simulink model "dcom_project"  (R2024b)
settings: Solver=VariableStepAuto  StartTime=0.0  StopTime=10.0  RelTol=1e-3
libraries: simulink x8, dspquant2 x8, dspfdesign x4, dspsigops x4, commdigbbndam3 x2
settings Model: Creator=HP  LastModifiedBy=HP

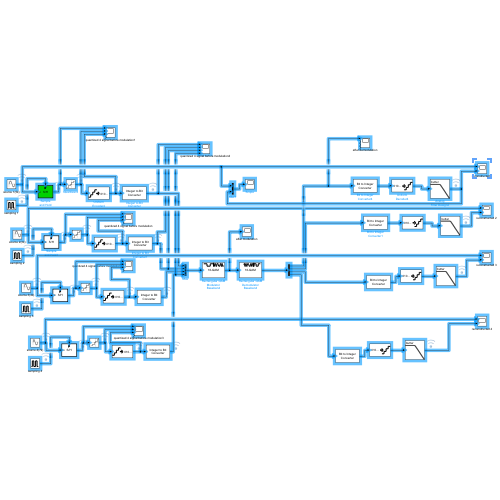
[thumbnail: Simulink's stored preview of the top-level diagram]
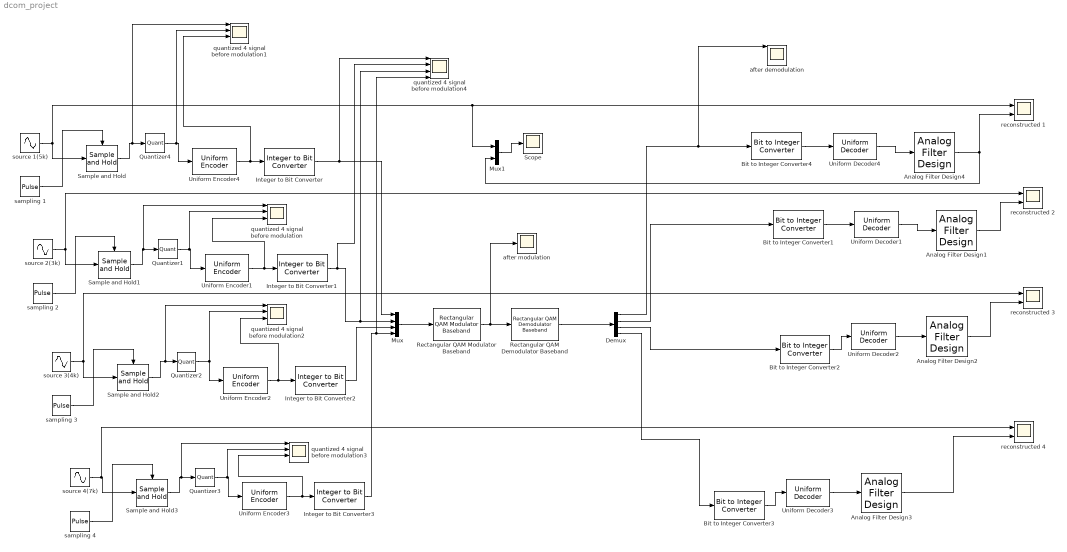
== system dcom_project ==
  Analog Filter Design1 : dspfdesign/Analog Filter Design  method=Butterworth  filttype=Lowpass  N=8  Wlo=2*pi*3000  Whi=80  Rp=2  Rs=40
  Analog Filter Design2 : dspfdesign/Analog Filter Design  method=Butterworth  filttype=Lowpass  N=8  Wlo=2*pi*4000  Whi=80  Rp=2  Rs=40
  Analog Filter Design3 : dspfdesign/Analog Filter Design  method=Butterworth  filttype=Lowpass  N=8  Wlo=2*pi*7000  Whi=80  Rp=2  Rs=40
  Analog Filter Design4 : dspfdesign/Analog Filter Design  method=Butterworth  filttype=Lowpass  N=8  Wlo=2*pi*5000  Whi=80  Rp=2  Rs=40
  Bit to Integer Converter{1..4} (4 alike) : simulink/Logic and Bit Operations/Bit to Integer Converter  nbits=4  bitOrder=MSB first  signedOutputValues=Signed  outDtype=Inherit via internal rule  outDtypeSigned=int8
      settings: LibrarySourceBlock=|
      | commutil2/Bit to Integer
      | Converter
  Demux : Demux
  Integer to Bit Converter{,1..3} (4 alike) : simulink/Logic and Bit Operations/Integer to Bit Converter  nbits=4  signedInputValues=Signed  bitOrder=MSB first  outDtype=Inherit via internal rule
      settings: LibrarySourceBlock=|
      | commutil2/Integer to Bit
      | Converter
  Mux : Mux
  Mux1 : Mux  Inputs=2
  Quantizer{1..4} (4 alike) : Quantizer  QuantizationInterval=0.125
  Rectangular QAM Demodulator Baseband : commdigbbndam3/Rectangular QAM Demodulator Baseband  M=16  OutType=Bit  DecType=Hard decision  VarSource=Dialog  Variance=1  Dec=Gray  Mapping=[0:15]  PowType=Min. distance between symbols  MinDist=2  AvgPow=1  PeakPow=1  Ph=0  outDtype1=Inherit via internal rule  outDtype2=Inherit via internal rule  derotateFactorWordLen=16  derotateFactorDataTypeStr=Inherit: Same word length as input  derotateFactorLastDataTypeStr=Inherit: Same word length as input  denormFactorWordLen=16  denormFactorDataTypeStr=Inherit: Same word length as input  denormFactorLastDataTypeStr=Inherit: Same word length as input  prodOutWordLen=32  prodOutOverflowMode=Wrap  prodOutRoundingMode=Floor  prodOutOvFlMode=off  prodOutOvFlModeLastStrValue=off  sumWordLen=32
      settings: LibrarySourceBlock=|
      | commhdldigbbndam/Rectangular QAM
      | Demodulator
      | Baseband
  Rectangular QAM Modulator Baseband : commdigbbndam3/Rectangular QAM Modulator Baseband  M=16  InType=Bit  Enc=Gray  Mapping=[0:15]  PowType=Min. distance between symbols  MinDist=2  AvgPow=1  PeakPow=1  Ph=0  outDtype=double  outWordLen=16  outUDDataType=sfix(16)  outFracLenMode=Best precision  outFracLen=15  outDataTypeStr=double  outLastDataTypeStr=double
      settings: LibrarySourceBlock=|
      | commhdldigbbndam/Rectangular QAM
      | Modulator
      | Baseband
  Sample and Hold{,1..3} (4 alike) : dspsigops/Sample and Hold  trig=Rising edge  initCond=0  latchinput=off
  Scope : Scope
  Uniform Decoder1 : dspquant2/Uniform Decoder  peak=5  bits=4  overflowMode=Saturate  otype=double
  Uniform Decoder2 : dspquant2/Uniform Decoder  peak=5  bits=4  overflowMode=Saturate  otype=double
  Uniform Decoder3 : dspquant2/Uniform Decoder  peak=5  bits=4  overflowMode=Saturate  otype=double
  Uniform Decoder4 : dspquant2/Uniform Decoder  peak=1.5  bits=4  overflowMode=Saturate  otype=double
  Uniform Encoder{1..4} (4 alike) : dspquant2/Uniform Encoder  peak=1.5  bits=4  otype=Signed integer
  after demodulation : Scope  NumInputPorts=4
  after modulation : Scope
  quantized 4 signal before modulation{,1..4} (5 alike) : Scope  NumInputPorts=4
  reconstructed {1..4} (4 alike) : Scope  NumInputPorts=2
  sampling 1 : DiscretePulseGenerator  PulseType=Time based  Period=1/40000  PulseWidth=50
  sampling 2 : DiscretePulseGenerator  PulseType=Time based  Period=1/24000  PulseWidth=50
  sampling 3 : DiscretePulseGenerator  PulseType=Time based  Period=1/32000  PulseWidth=50
  sampling 4 : DiscretePulseGenerator  PulseType=Time based  Period=1/56000  PulseWidth=50
  source 1(5k) : Sin  Frequency=2*pi*5000  Phase=pi/2  SampleTime=0
  source 2(3k) : Sin  Frequency=2*pi*3000  Phase=pi/2  SampleTime=0
  source 3(4k) : Sin  Frequency=2*pi*4000  Phase=pi/2  SampleTime=0
  source 4(7k) : Sin  Frequency=2*pi*7000  Phase=pi/2  SampleTime=0
  wires:
  sampling 1/1 -> Sample and Hold/Trigger
  Sample and Hold/1 -> quantized 4 signal before modulation1/1, Quantizer4/1
  Quantizer4/1 -> quantized 4 signal before modulation1/2, Uniform Encoder4/1
  Uniform Encoder4/1 -> quantized 4 signal before modulation1/3, Integer to Bit Converter/1
  Sample and Hold1/1 -> quantized 4 signal before modulation/1, Quantizer1/1
  Uniform Encoder1/1 -> quantized 4 signal before modulation/3, Integer to Bit Converter1/1
  sampling 2/1 -> Sample and Hold1/Trigger
  Quantizer1/1 -> quantized 4 signal before modulation/2, Uniform Encoder1/1
  Uniform Decoder1/1 -> Analog Filter Design1/1
  Bit to Integer Converter1/1 -> Uniform Decoder1/1
  source 2(3k)/1 -> Sample and Hold1/1, reconstructed 2/1
  Sample and Hold2/1 -> quantized 4 signal before modulation2/1, Quantizer2/1
  Uniform Encoder2/1 -> quantized 4 signal before modulation2/3, Integer to Bit Converter2/1
  sampling 3/1 -> Sample and Hold2/Trigger
  Quantizer2/1 -> quantized 4 signal before modulation2/2, Uniform Encoder2/1
  Uniform Decoder2/1 -> Analog Filter Design2/1
  Bit to Integer Converter2/1 -> Uniform Decoder2/1
  source 3(4k)/1 -> Sample and Hold2/1, reconstructed 3/1
  Analog Filter Design2/1 -> reconstructed 3/2
  Sample and Hold3/1 -> quantized 4 signal before modulation3/1, Quantizer3/1
  Uniform Encoder3/1 -> quantized 4 signal before modulation3/3, Integer to Bit Converter3/1
  sampling 4/1 -> Sample and Hold3/Trigger
  Quantizer3/1 -> quantized 4 signal before modulation3/2, Uniform Encoder3/1
  Uniform Decoder3/1 -> Analog Filter Design3/1
  Bit to Integer Converter3/1 -> Uniform Decoder3/1
  Analog Filter Design3/1 -> reconstructed 4/2
  Integer to Bit Converter/1 -> quantized 4 signal before modulation4/1, Mux/1
  Integer to Bit Converter2/1 -> Mux/3
  Mux/1 -> Rectangular QAM Modulator Baseband/1
  Integer to Bit Converter3/1 -> quantized 4 signal before modulation4/4, Mux/4
  Bit to Integer Converter4/1 -> Uniform Decoder4/1
  Uniform Decoder4/1 -> Analog Filter Design4/1
  Demux/1 -> after demodulation/1, Bit to Integer Converter4/1
  Demux/2 -> Bit to Integer Converter1/1
  Demux/3 -> Bit to Integer Converter2/1
  Demux/4 -> Bit to Integer Converter3/1
  Rectangular QAM Demodulator Baseband/1 -> Demux/1
  Analog Filter Design1/1 -> reconstructed 2/2
  Analog Filter Design4/1 -> Mux1/2, reconstructed 1/2
  source 1(5k)/1 -> Sample and Hold/1, Mux1/1, reconstructed 1/1
  Rectangular QAM Modulator Baseband/1 -> Rectangular QAM Demodulator Baseband/1, after modulation/1
  source 4(7k)/1 -> reconstructed 4/1, Sample and Hold3/1
  Integer to Bit Converter1/1 -> quantized 4 signal before modulation4/2, quantized 4 signal before modulation4/3, Mux/2
  Mux1/1 -> Scope/1
